simulink model "actuator_control"  (R2015a)
settings: Solver=FixedStepDiscrete  StartTime=0.0  StopTime=inf  FixedStep=sample_time  RelTol=1e-3
undefined symbols (not defined in the file): A_kalman_swing_load, A_lpf_dtau, B1_lpf_dtau, B2_lpf_dtau, B_kalman_swing_load, C_kalman_swing_load, Discrete, fdesignblkfcn, gcbh, initial_dx_estimate, j_segments, k_sea_low, lateral_motor_efficiency, P0_kalman_swing_load, sample_time, swing_collision_damping_rate, Time
libraries: simulink x11, dsparch4 x6, ctrlSharedLib x4, dspfdesign x2
(part 2 of 2)

== matlab function actuator_control/Load Torque Kalman Filter/MATLAB Function ==
  data: spring_torques input; R1 output; sample_time parameter; R2 output; R3 output; R4 output
function [R1, R2, R3, R4] = MeasurementCovariance(spring_torques, sample_time)
         
    high_torque_threshold = 80;
    low_torque_threshold = 50;
    high_deviation = 10;
    low_deviation = 0.1;
    
    deviation = (abs(spring_torques)-low_torque_threshold)*(low_deviation-high_deviation)/(high_torque_threshold-low_torque_threshold) + high_deviation;
    deviation(abs(spring_torques) <= low_torque_threshold) = high_deviation;
    deviation(abs(spring_torques) >= high_torque_threshold) = low_deviation;

    R1 = diag([(1e-6)^2, deviation(1)^2])/sample_time;
    R2 = diag([(1e-6)^2, deviation(2)^2])/sample_time;
    R3 = diag([(1e-6)^2, deviation(3)^2])/sample_time;
    R4 = diag([(1e-6)^2, deviation(4)^2])/sample_time;
end

== matlab function actuator_control/Detect Collision ==
  data: time input; spring_torque input; load_torque_derivative input; in_collision output; swing_collision_wait_time parameter
function in_collision = detect_collision(time, spring_torque, load_torque_derivative, swing_collision_wait_time)
    
    persistent collision_state time_of_collision;
    if isempty(collision_state)
        collision_state = logical(zeros(4,1));
        time_of_collision = zeros(4,1);
    end

    collision_detected = (abs(load_torque_derivative) > 2000 | abs(spring_torque) >= 50) & (time - time_of_collision > (1.5*swing_collision_wait_time));
    time_of_collision(collision_detected) = time;
    collision_state = collision_state | collision_detected;
    time_since_collision = time - time_of_collision;
    out_of_collision = (time_since_collision > swing_collision_wait_time) & (abs(spring_torque) < 50);
    collision_state(out_of_collision) = 0;
    %in_collision = collision_state;
    in_collision = [collision_state(1) | collision_state(2);
                    collision_state(1) | collision_state(2);
                    collision_state(3) | collision_state(4);
                    collision_state(3) | collision_state(4)];
    
end

== matlab function actuator_control/SEA Controller (Velocity)/Nonlinear Spring Force ==
  data: deflections input; tau_sea output
function tau_sea   = SeaSpringForce( deflections )
    tau_sea = SeaSpringForce( deflections );
end

== matlab function actuator_control/Load Motion Disturbance Observer (Swing) Error-Proportional - 2nd order ==
  data: reset input; spring_torques input; d_hat_tp1 output size=[1 4]; positions input; velocities input; j_segments parameter; sample_time parameter
function d_hat_tp1  = disturbance_observer(reset, spring_torques, positions, velocities, j_segments, sample_time)

    order = 2;
    L = 2*2.^[1:order+1] .* factorial(order+1)./(factorial(order+1-(1:(order+1))).*factorial(1:order+1));
    N = 4;
    
    persistent z_t d_hat_t integral_term;
    if isempty(z_t)
        z_t = zeros(1,N);
        d_hat_t = zeros(1,N);
        integral_term = zeros(order,N);
    end
    
    for i=1:N
        if reset(i)
            z_t(i) = 0;
            d_hat_t(i) = 0;
            integral_term(:,i) = 0;
        end
    end
   
    % Define system
    A_d = [1, sample_time; 0, 1];
    Bu_d = [zeros(1,N); sample_time./j_segments];
    A_c = [0 1; 0 0];
    Bu_c = [zeros(1,N); 1./j_segments];
    Bd_c = [zeros(1,N); 1./j_segments];
    x = [positions'; velocities'];
    u = spring_torques;
 
    % Estimate disturbances
    z_tp1 = zeros(1,N);
    x_tp1 = zeros(2,N);
    d_hat_tp1 = zeros(1,N);
    for i=1:N
        z_tp1(i) = z_t(i) + sample_time*(pinv(Bd_c(:,i))*(A_c*x(:,i) + Bu_c(:,i)*u(i)) + d_hat_t(i));
        x_tp1(:,i) = A_d*x(:,i) + Bu_d(:,i)*u(i);
        integral_term(1,i) = integral_term(1,i) + sample_time*(pinv(Bd_c(:,i))*x_tp1(:,i) - z_tp1(i));
        for j=2:order
            integral_term(j,i) = integral_term(j,i) + sample_time*integral_term(j-1,i);
        end
        d_hat_tp1(i) = L*[(pinv(Bd_c(:,i))*x_tp1(:,i) - z_tp1(i)); integral_term(:,i)];
        d_hat_t(i) = d_hat_tp1(i);
        z_t(i) = z_tp1(i);
    end
    
end
